simulink subsystem "Interpolate"  (R2022a)
settings: Solver=VariableStepAuto  StartTime=0.0  StopTime=10.0  RelTol=1e-3
settings Model: Creator=bkfre  LastModifiedBy=bkfre

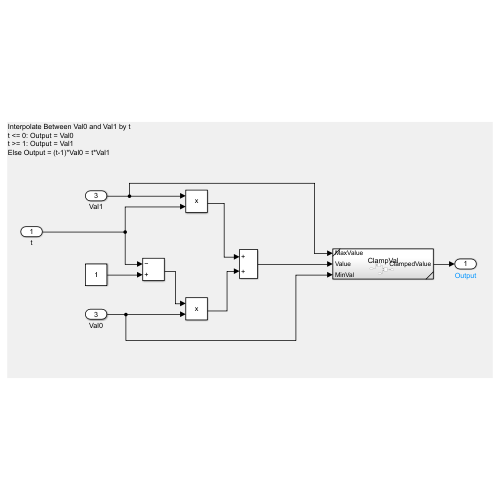
[thumbnail: Simulink's stored preview of the top-level diagram]
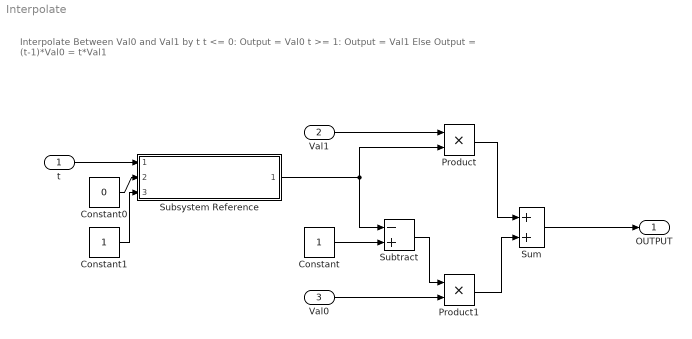
== system Interpolate ==
  note: Interpolate Between Val0 and Val1 by t
      | t <= 0: Output = Val0
      | t >= 1: Output = Val1
      | Else Output = (t-1)*Val0 = t*Val1
  t : Inport
  Val1 : Inport  Port=2
  Val0 : Inport  Port=3
  Constant : Constant
  Constant0 : Constant  Value=0
  Constant1 : Constant
  Product : Product
  Product1 : Product
  Subsystem Reference : Subsystem  ReferencedSubsystem=ClampVal
  Subtract : Sum  Inputs=-+
  Sum : Sum
  OUTPUT : Outport
  wires:
  Sum/1 -> OUTPUT/1
  Val0/1 -> Product1/2
  Subtract/1 -> Product1/1
  Product1/1 -> Sum/2
  Product/1 -> Sum/1
  Constant/1 -> Subtract/2
  Subsystem Reference/1 -> Product/2, Subtract/1
  Val1/1 -> Product/1
  t/1 -> Subsystem Reference/1
  Constant1/1 -> Subsystem Reference/3
  Constant0/1 -> Subsystem Reference/2
